simulink model "3_phase_squirrel_cage"  (R2024a)
settings: Solver=VariableStepAuto  StartTime=0.0  StopTime=3  RelTol=1e-3
libraries: spsACVoltageSourceLib x3, spsAsynchronousMachineSIUnitsLib x1, spsGroundLib x1, sps_lib x1
settings Model: Creator=baileyraven  LastModifiedBy=baileyraven
settings OptimizationCC: ReuseModelBlockBuffer=off
settings RTWCC: GPUComputeCapability=3.5

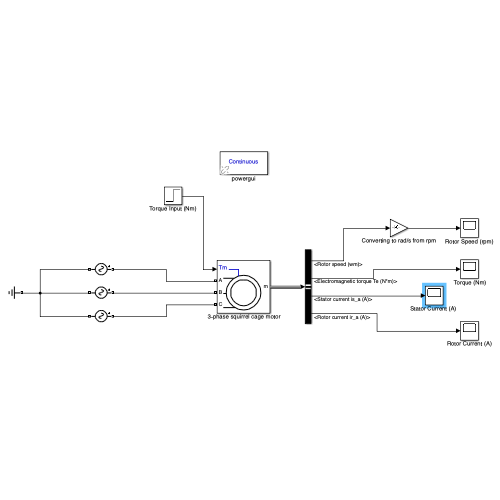
[thumbnail: Simulink's stored preview of the top-level diagram]
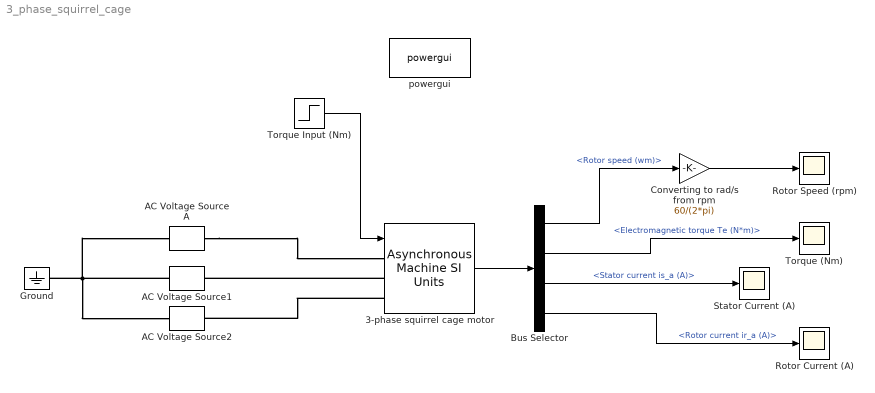
== system 3_phase_squirrel_cage ==
  " 3-phase squirrel cage motor" : spsAsynchronousMachineSIUnitsLib/Asynchronous Machine SI Units  RotorType=Squirrel-cage  PresetModel=No  MechanicalLoad=Torque Tm  ShowDetailedParameters=on  ReferenceFrame=Rotor  Units=SI  MeasurementBus=off  NominalParameters=[7460 281.69 50]  VoltageRatio=1  Stator=[0.8 0.009063]  Rotor=[0.8 0.009063]  Cage1=[0.4155 0.002066]  Cage2=[0.4168 0.0003495]  Lm=0.637  Mechanical=[0.1 0 2]  PolePairs=2  InitialConditions=[1 0 0 0 0 0 0 0]  SimulateSaturation=off  Saturation=[14.03593122, 27.81365428, 53.79336849, 72.68890987, 97.98006896, 148.6815601, 215.7428561, 302.9841135, 428.7778367 ; 230, 322, 414, 460, 506, 552, 598, 644, 690]  LoadFlowParameters=1492000  TsPowergui=0  TsBlock=-1  IterativeModel=Trapezoidal non iterative  IterativeDiscreteModel=Trapezoidal non iterative  Pmec=1.492e+006
  " Torque (Nm)" : Scope
  AC Voltage Source A : spsACVoltageSourceLib/AC Voltage Source  Amplitude=325.269  Phase=0  Frequency=50  SampleTime=0  Measurements=None  BusType=swing  Pref=10e3  Qref=0  Qmin=-inf  Qmax=+inf
  AC Voltage Source1 : spsACVoltageSourceLib/AC Voltage Source  Amplitude=325.369  Phase=-120  Frequency=50  SampleTime=0  Measurements=None  BusType=swing  Pref=10e3  Qref=0  Qmin=-inf  Qmax=+inf
  AC Voltage Source2 : spsACVoltageSourceLib/AC Voltage Source  Amplitude=325.269  Phase=-240  Frequency=50  SampleTime=0  Measurements=None  BusType=swing  Pref=10e3  Qref=0  Qmin=-inf  Qmax=+inf
  Bus Selector : BusSelector  OutputSignals=Mechanical.Rotor speed (wm),Mechanical.Electromagnetic torque Te (N*m),Stator measurements.Stator current is_a (A),Rotor measurements.Rotor current ir_a (A)
  Converting to rad/s from rpm : Gain  Gain=60/(2*pi)
  Ground : spsGroundLib/Ground  LConnTagsString=a
  Rotor Current (A) : Scope
  Rotor Speed (rpm) : Scope
  "Stator Current (A) " : Scope
  Torque Input (Nm) : Step  Time=1.5  After=49.89  SampleTime=0
  powergui : sps_lib/powergui  Priority=1  SimulationMode=Continuous  SampleTime=50e-6  frequency=60  Iterations=50  frequencyindice=50  Pbase=100e6  ErrMax=1e-4  UnitsV=kV  UnitsW=MW  buscounter=0  FunctionMessages=off  echomessages=off  EnableUseOfTLC=off  CurrentSourceSwitches=off  DisableSnubberDevices=off  DisableRonSwitches=off  DisableVfSwitches=off  DisplayEquations=off  AutomaticDiscreteSolvers=off  SolverType=Tustin/Backward Euler (TBE)  Interpol=off  ExternalGateDelay=off  methode=off  Ts=100  x0status=blocks  SPID=on  SwTol=0  HookPort=off  NonlinearTolerance=1e-4  nMaxIteration=100  ContinueOnMaxIteration=off  RestoreLinks=warning  ResistiveCurrentMeasurement=off  Frange=[0:2:500]  Ylog=off  Xlog=on  ShowGrid=off  save=off  variable=ZData  structure=0  ZoomFFT=off  StartTime=0.0  cycles=1  DisplayStyle=1  fundamental=60  FreqAxis=off  MaxFrequency=1000  frequencyindicesteady=1  RmsSteady=1  display=off
  wires:
  " 3-phase squirrel cage motor"/1 -> Bus Selector/1
  Torque Input (Nm)/1 -> " 3-phase squirrel cage motor"/1
  Bus Selector/2 -> " Torque (Nm)"/1  "<Electromagnetic torque Te (N*m)>"
  Bus Selector/3 -> "Stator Current (A) "/1  "<Stator current is_a (A)>"
  Bus Selector/4 -> Rotor Current (A)/1  "<Rotor current ir_a (A)>"
  Bus Selector/1 -> Converting to rad/s from rpm/1  "<Rotor speed (wm)>"
  Converting to rad/s from rpm/1 -> Rotor Speed (rpm)/1
  connections:
  Ground/LConn1 -- AC Voltage Source2/LConn1 -- AC Voltage Source1/LConn1 -- AC Voltage Source A/LConn1
  " 3-phase squirrel cage motor"/LConn2 -- AC Voltage Source1/RConn1
  AC Voltage Source A/RConn1 -- " 3-phase squirrel cage motor"/LConn1
  " 3-phase squirrel cage motor"/LConn3 -- AC Voltage Source2/RConn1
